simulink library "calcDistanceFromPath_new"  (R2020a)
settings: Solver=VariableStepAuto  StartTime=0.0  StopTime=10.0  RelTol=1e-3
libraries: calculate_vector_magnitude x1, pathGeometry_ul x1
settings Model: Creator=Ayaz  LastModifiedBy=Ayaz

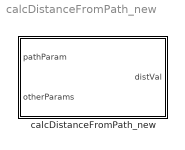
== system calcDistanceFromPath_new ==
  calcDistanceFromPath_new : Subsystem

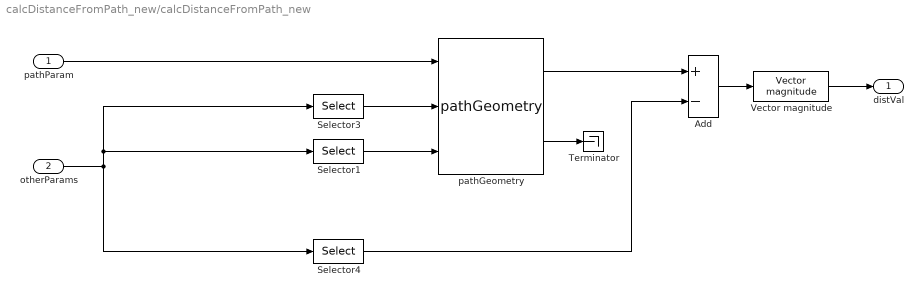
== system calcDistanceFromPath_new/calcDistanceFromPath_new ==
  pathParam : Inport
  otherParams : Inport  Port=2
  Add : Sum  Inputs=+-
  Selector1 : Selector  InputPortWidth=11  IndexOptions=Index vector (dialog)  Indices=6:8  OutputSizes=1
  Selector3 : Selector  InputPortWidth=11  IndexOptions=Index vector (dialog)  Indices=1:5  OutputSizes=1
  Selector4 : Selector  InputPortWidth=11  IndexOptions=Index vector (dialog)  Indices=9:11  OutputSizes=1
  Terminator : Terminator
  Vector magnitude : calculate_vector_magnitude/Vector magnitude  SystemSampleTime=-1  Latency=0  AutoFrameSizeCalculation=off
  pathGeometry : pathGeometry_ul/pathGeometry  SystemSampleTime=-1  Latency=0  AutoFrameSizeCalculation=off
  distVal : Outport
  wires:
  Vector magnitude/1 -> distVal/1
  otherParams/1 -> Selector1/1, Selector3/1, Selector4/1
  pathParam/1 -> pathGeometry/1
  Selector3/1 -> pathGeometry/2
  pathGeometry/1 -> Add/1
  Selector4/1 -> Add/2
  Add/1 -> Vector magnitude/1
  Selector1/1 -> pathGeometry/3
  pathGeometry/2 -> Terminator/1
